simulink model "controller"  (R2022a)
settings: Solver=VariableStepAuto  StartTime=0.0  StopTime=10.0  RelTol=1e-3
settings Model: Creator=mheubach  LastModifiedBy=mheubach

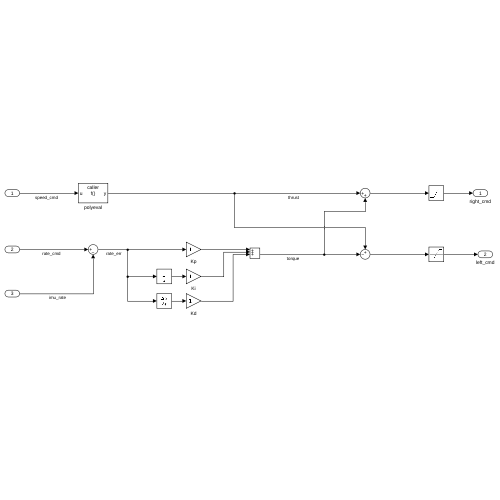
[thumbnail: Simulink's stored preview of the top-level diagram]
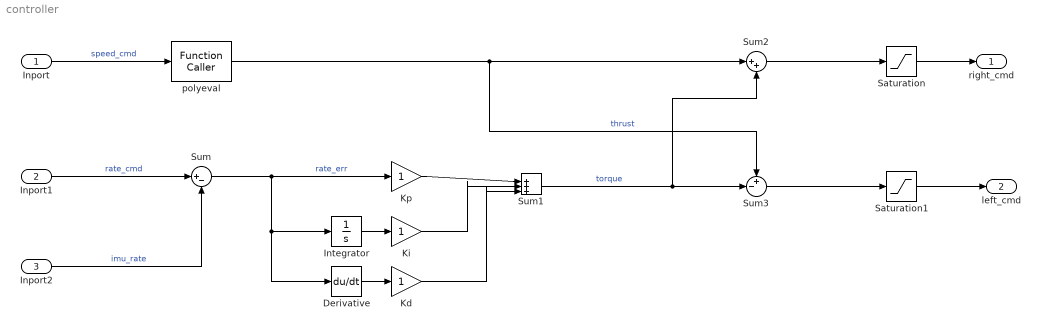
== system controller ==
  Inport : Inport
  Inport1 : Inport  Port=2
  Inport2 : Inport  Port=3
  Derivative : Derivative
  Integrator : Integrator
  Kd : Gain
  Ki : Gain
  Kp : Gain
  Saturation : Saturate
  Saturation1 : Saturate
  Sum : Sum  Inputs=|+-
  Sum1 : Sum  Inputs=+++|
  Sum2 : Sum  Inputs=|++
  Sum3 : Sum  Inputs=+-|
  polyeval : FunctionCaller  FunctionPrototype=y = f(u)  InputArgumentSpecifications=<Enter example>  OutputArgumentSpecifications=<Enter example>
  right_cmd : Outport
  left_cmd : Outport  Port=2
  wires:
  Inport/1 -> polyeval/1  "speed_cmd"
  Inport1/1 -> Sum/1  "rate_cmd"
  Inport2/1 -> Sum/2  "imu_rate"
  Integrator/1 -> Ki/1
  Derivative/1 -> Kd/1
  Sum/1 -> Kp/1, Integrator/1, Derivative/1  "rate_err"
  Kp/1 -> Sum1/1
  Ki/1 -> Sum1/2
  Kd/1 -> Sum1/3
  Sum1/1 -> Sum3/2, Sum2/2  "torque"
  Sum3/1 -> Saturation1/1
  polyeval/1 -> Sum2/1, Sum3/1  "thrust"
  Sum2/1 -> Saturation/1
  Saturation1/1 -> left_cmd/1
  Saturation/1 -> right_cmd/1
